simulink model "final"  (R2015b)
settings: Solver=VariableStepAuto  StartTime=0.0  StopTime=10.0  RelTol=1e-3
libraries: simulink_extras x2, dsparch4 x1, commsynccomp2 x1, rfmathmodels1 x1, dspsigops x1
settings Model: Creator=dimple  LastModifiedBy=dimple

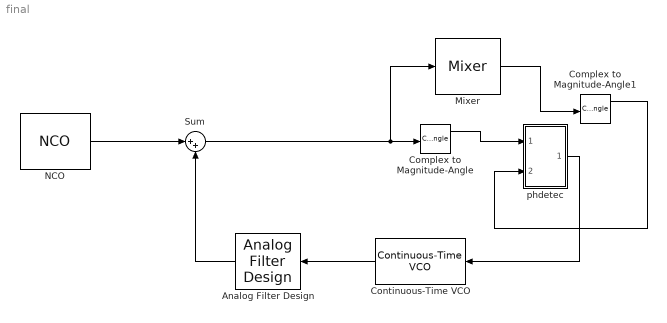
== system final ==
  Analog Filter Design : dsparch4/Analog Filter Design  method=Butterworth  filttype=Lowpass  N=5  Wlo=1e6*2*pi  Whi=80  Rp=2  Rs=40
  Complex to Magnitude-Angle : ComplexToMagnitudeAngle
  Complex to Magnitude-Angle1 : ComplexToMagnitudeAngle
  Continuous-Time VCO : commsynccomp2/Continuous-Time VCO  Ac=1  Fc=1e6  Kc=1e5  Ph=0
  Mixer : rfmathmodels1/Mixer  gain=0  PhNs=-120  Fo=100  seed=2137  loss=0
  NCO : dspsigops/NCO  AccIncSrc=Specify via dialog  AccInc=100  PhaseOffsetSrc=Specify via dialog  PhaseOffset=0  AccumWL=16  HasDither=on  DitherWL=4  PNgeneratorLength=19  HasPhaseQuantizer=on  TableDepth=12  HasOutputPhaseError=off  Formula=Complex exponential  DataType=double  OutputWL=16  OutputFL=14  CompMethod=Table lookup (no interpolation)  SampleTime=1  SamplesPerFrame=1  OutputFrames=off
  Sum : Sum  Inputs=|++
  "phdetec " : Subsystem
  wires:
  NCO/1 -> Sum/1
  Sum/1 -> Complex to Magnitude-Angle/1, Mixer/1
  Continuous-Time VCO/1 -> Analog Filter Design/1
  Analog Filter Design/1 -> Sum/2
  Complex to Magnitude-Angle/1 -> "phdetec "/1(In1)
  "phdetec "/1("Out ") -> Continuous-Time VCO/1
  Mixer/1 -> Complex to Magnitude-Angle1/1
  Complex to Magnitude-Angle1/1 -> "phdetec "/2(In2)

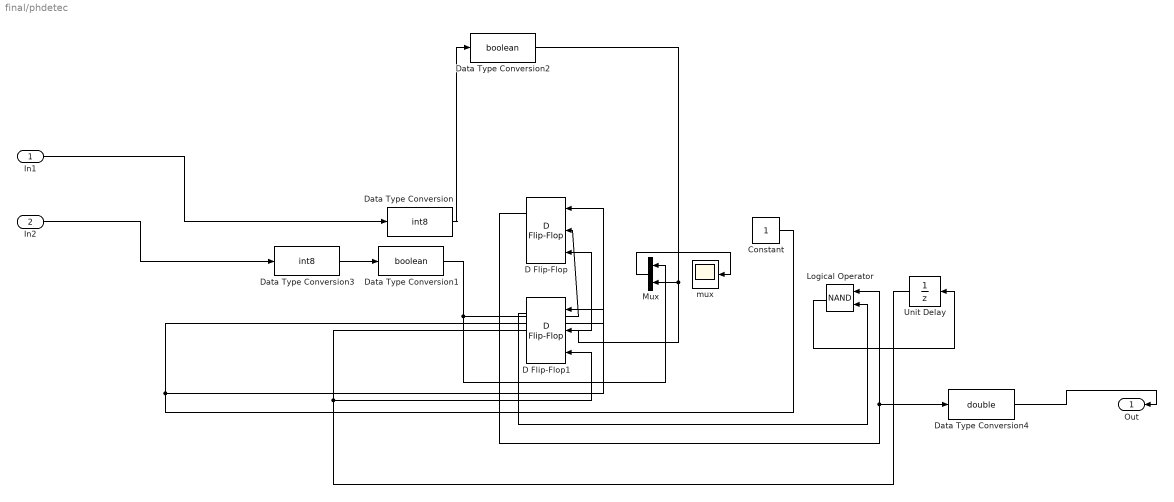
== system final/phdetec  ==
  In1 : Inport
  In2 : Inport  Port=2
  Constant : Constant  OutDataTypeStr=boolean
  D Flip-Flop : simulink_extras/Flip Flops/D Flip-Flop
  D Flip-Flop1 : simulink_extras/Flip Flops/D Flip-Flop
  Data Type Conversion : DataTypeConversion  OutDataTypeStr=int8
  Data Type Conversion1 : DataTypeConversion  OutDataTypeStr=boolean
  Data Type Conversion2 : DataTypeConversion  OutDataTypeStr=boolean
  Data Type Conversion3 : DataTypeConversion  OutDataTypeStr=int8
  Data Type Conversion4 : DataTypeConversion  OutDataTypeStr=double
  Logical Operator : Logic  Operator=NAND  AllPortsSameDT=off  OutDataTypeStr=boolean
  Mux : Mux  Inputs=2
  Unit Delay : UnitDelay  SampleTime=0.01
  "mux " : Scope
  "Out " : Outport
  wires:
  Data Type Conversion1/1 -> D Flip-Flop/2, Mux/1
  D Flip-Flop1/1 -> Logical Operator/2
  D Flip-Flop/1 -> Logical Operator/1, Data Type Conversion4/1
  In2/1 -> Data Type Conversion3/1
  Constant/1 -> D Flip-Flop/1, D Flip-Flop1/1
  Mux/1 -> "mux "/1
  Logical Operator/1 -> Unit Delay/1
  Unit Delay/1 -> D Flip-Flop/3, D Flip-Flop1/3
  Data Type Conversion2/1 -> D Flip-Flop1/2, Mux/2
  Data Type Conversion3/1 -> Data Type Conversion1/1
  In1/1 -> Data Type Conversion/1
  Data Type Conversion/1 -> Data Type Conversion2/1
  Data Type Conversion4/1 -> "Out "/1
